simulink model "Work_demo"  (R2022b)
settings: Solver=VariableStepAuto  StartTime=0.0  StopTime=10.0  RelTol=1e-3
libraries: fl_lib x19, nesl_utility x6
(part 2 of 2)

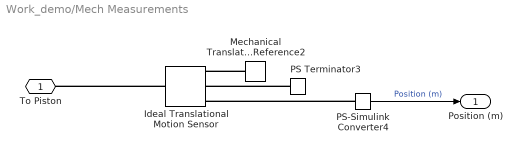
== system Work_demo/Mech Measurements ==
  Ideal Translational Motion Sensor : fl_lib/Mechanical/Mechanical Sensors/Ideal Translational Motion Sensor  reference=foundation.enum.MeasurementReference.difference  acceleration_port=false  velocity_port=true  position_port=true  offset=0 m
  Mechanical Translational Reference2 : fl_lib/Mechanical/Translational Elements/Mechanical Translational Reference
  PS Terminator3 : fl_lib/Physical Signals/Sinks/PS Terminator
  PS-Simulink Converter4 : nesl_utility/PS-Simulink Converter  PhysicalDomain=network_engine_domain  SubClassName=ps_output  LeftPortType=input  RightPortType=output  PseudoPeriodic=off  Frequencies=[]  VectorFormat=inherit  Unit=m  AffineConversion=off
  "To Piston " : PMIOPort  Side=Left
  Position (m) : Outport
  wires:
  PS-Simulink Converter4/1 -> Position (m)/1  "Position (m)"
  connections:
  Mechanical Translational Reference2/LConn1 -- Ideal Translational Motion Sensor/RConn1
  PS-Simulink Converter4/LConn1 -- Ideal Translational Motion Sensor/RConn3
  PS Terminator3/LConn1 -- Ideal Translational Motion Sensor/RConn2
  Ideal Translational Motion Sensor/LConn1 -- "To Piston "/RConn1

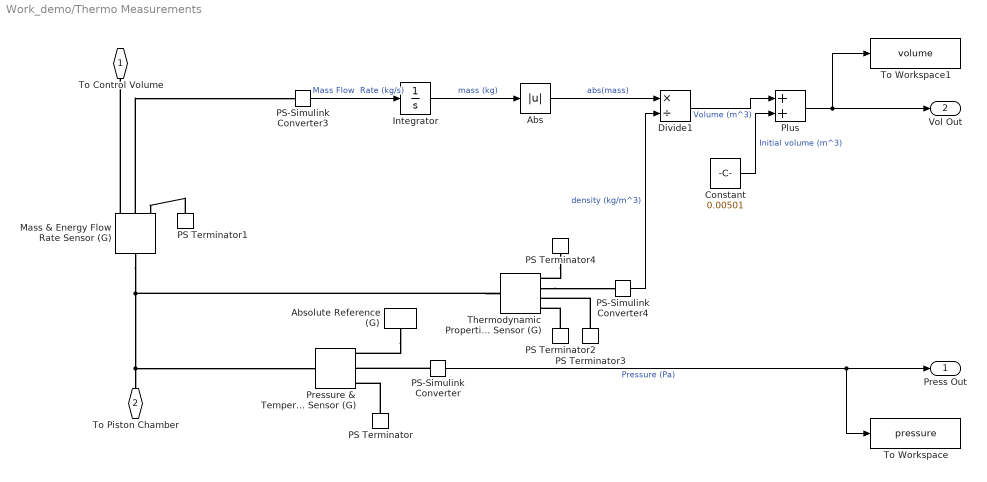
== system Work_demo/Thermo Measurements ==
  Abs : Abs  SaturateOnIntegerOverflow=off
  Absolute Reference (G) : fl_lib/Gas/Elements/Absolute Reference (G)
      settings: InternalSimscapePortConfiguration="{\"Bottom\":[],\"Left\":[{\"id\":\"A\",\"label\":\"\",\"type\":\"foundation.gas.gas\"}],\"Right\":[],\"Top\":[]}"
  Constant : Constant  Value=0.00501
  Divide1 : Product  Inputs=*/
  Integrator : Integrator
  Mass & Energy Flow Rate Sensor (G) : fl_lib/Gas/Sensors/Mass & Energy Flow Rate Sensor (G)
      settings: InternalSimscapePortConfiguration="{\"Bottom\":[],\"Left\":[{\"id\":\"A\",\"label\":\"A\",\"type\":\"foundation.gas.gas\"}],\"Right\":[{\"id\":\"B\",\"label\":\"B\",\"type\":\"foundation.gas.gas\"},{\"id\":\"M\",\"label\":\"M\",\"type\":\"output\"},{\"id\":\"PHI\",\"label\":\"Phi\",\"type\":\"output\"}],\"Top\":[]}"
  PS Terminator{,1..4} (5 alike) : fl_lib/Physical Signals/Sinks/PS Terminator
  PS-Simulink Converter : nesl_utility/PS-Simulink Converter  PhysicalDomain=network_engine_domain  SubClassName=ps_output  LeftPortType=input  RightPortType=output  PseudoPeriodic=off  Frequencies=[]  VectorFormat=inherit  Unit=Pa  AffineConversion=off
  PS-Simulink Converter3 : nesl_utility/PS-Simulink Converter  PhysicalDomain=network_engine_domain  SubClassName=ps_output  LeftPortType=input  RightPortType=output  PseudoPeriodic=off  Frequencies=[]  VectorFormat=inherit  Unit=kg/s  AffineConversion=off
  PS-Simulink Converter4 : nesl_utility/PS-Simulink Converter  PhysicalDomain=network_engine_domain  SubClassName=ps_output  LeftPortType=input  RightPortType=output  PseudoPeriodic=off  Frequencies=[]  VectorFormat=inherit  Unit=kg/m^3  AffineConversion=off
  Plus : Sum
  Pressure & Temperature Sensor (G) : fl_lib/Gas/Sensors/Pressure & Temperature Sensor (G)
      settings: InternalSimscapePortConfiguration="{\"Bottom\":[],\"Left\":[{\"id\":\"A\",\"label\":\"A\",\"type\":\"foundation.gas.gas\"}],\"Right\":[{\"id\":\"B\",\"label\":\"B\",\"type\":\"foundation.gas.gas\"},{\"id\":\"P\",\"label\":\"P\",\"type\":\"output\"},{\"id\":\"T\",\"label\":\"T\",\"type\":\"output\"}],\"Top\":[]}"
  Thermodynamic Properties Sensor (G) : fl_lib/Gas/Sensors/Thermodynamic Properties Sensor (G)  s_std=3.8635 kJ/(K*kg)  p_std=0.101325 MPa  T_std=293.15 K
      settings: InternalSimscapePortConfiguration="{\"Bottom\":[],\"Left\":[{\"id\":\"A\",\"label\":\"A\",\"type\":\"foundation.gas.gas\"}],\"Right\":[{\"id\":\"H\",\"label\":\"h\",\"type\":\"output\"},{\"id\":\"RHO\",\"label\":\"rho\",\"type\":\"output\"},{\"id\":\"CP\",\"label\":\"cp\",\"type\":\"output\"},{\"id\":\"S\",\"label\":\"s\",\"type\":\"output\"}],\"Top\":[]}"
  To Workspace : ToWorkspace  VariableName=pressure  SaveFormat=Timeseries  SampleTime=-1
  To Workspace1 : ToWorkspace  VariableName=volume  SaveFormat=Timeseries  SampleTime=-1
      settings: Save2DSignal=2-D array (concatenate along first dimension)
  To Control Volume : PMIOPort  Side=Left
  To Piston Chamber : PMIOPort  Port=2  Side=Left
  Press Out : Outport
  Vol Out : Outport  Port=2
  wires:
  Integrator/1 -> Abs/1  "mass (kg)"
  PS-Simulink Converter3/1 -> Integrator/1  "Mass Flow  Rate (kg/s)"
  Abs/1 -> Divide1/1  "abs(mass)"
  PS-Simulink Converter4/1 -> Divide1/2  "density (kg/m^3)"
  PS-Simulink Converter/1 -> To Workspace/1, Press Out/1  "Pressure (Pa)"
  Divide1/1 -> Plus/1  "Volume (m^3)"
  Plus/1 -> Vol Out/1, To Workspace1/1
  Constant/1 -> Plus/2  "Initial volume (m^3)"
  connections:
  PS-Simulink Converter/LConn1 -- Pressure & Temperature Sensor (G)/RConn2
  Mass & Energy Flow Rate Sensor (G)/LConn1 -- Thermodynamic Properties Sensor (G)/LConn1 -- To Piston Chamber/RConn1 -- Pressure & Temperature Sensor (G)/LConn1
  Mass & Energy Flow Rate Sensor (G)/RConn2 -- PS-Simulink Converter3/LConn1
  Absolute Reference (G)/LConn1 -- Pressure & Temperature Sensor (G)/RConn1
  Mass & Energy Flow Rate Sensor (G)/RConn1 -- To Control Volume/RConn1
  Thermodynamic Properties Sensor (G)/RConn2 -- PS-Simulink Converter4/LConn1
  PS Terminator/LConn1 -- Pressure & Temperature Sensor (G)/RConn3
  PS Terminator1/LConn1 -- Mass & Energy Flow Rate Sensor (G)/RConn3
  PS Terminator2/LConn1 -- Thermodynamic Properties Sensor (G)/RConn4
  PS Terminator3/LConn1 -- Thermodynamic Properties Sensor (G)/RConn3
  PS Terminator4/LConn1 -- Thermodynamic Properties Sensor (G)/RConn1
